simulink model "FOC_tune"  (R2022b)
settings: Solver=VariableStepAuto  StartTime=0.0  StopTime=40  RelTol=1e-3
libraries: spsMosfetLib x6, slpidlib x5, spsDCVoltageSourceLib x1, spsTriangleGeneratorLib x1, spsPermanentMagnetSynchronousMachineLib x1, spspowerguiLib x1
settings Model: Creator=ozgur  LastModifiedBy=ozgur

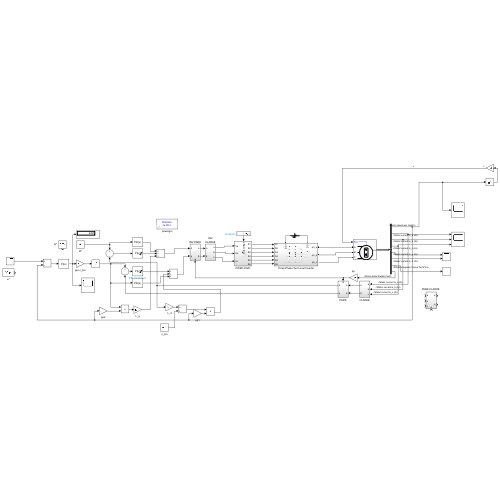
[thumbnail: Simulink's stored preview of the top-level diagram]
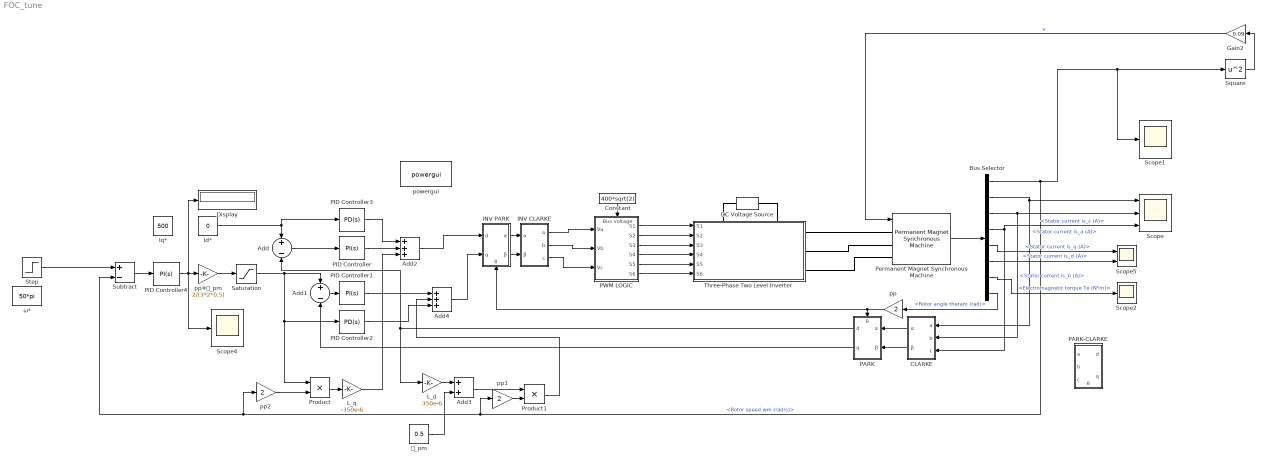
== system FOC_tune ==
  Add : Sum  Inputs=+-
  Add1 : Sum  Inputs=+-
  Add2 : Sum  Inputs=+++
  Add3 : Sum
  Add4 : Sum  Inputs=+++
  Bus Selector : BusSelector  OutputSignals=Rotor speed wm (rad/s),Stator current is_a (A),Stator current is_b (A),Stator current is_c (A),Stator current is_q (A),Stator current is_d (A),Electromagnetic torque Te (N*m),Rotor angle thetam (rad)
  CLARKE : Subsystem
  Constant : Constant  Value=400*sqrt(2)
  DC Voltage Source : spsDCVoltageSourceLib/DC Voltage Source  Amplitude=400*sqrt(2)  Measurements=None
  Display : Display
  Gain2 : Gain  Gain=0.09
  INV CLARKE : Subsystem
  INV PARK : Subsystem
      settings: PortSchema="{\"entries\":[{\"content\":{\"sides\":[{\"content\":{\"connectorIds\":[\"In1\",\"In2\"]},\"type\":\"ConnectorPlacement.EquallySpacedRectSide\",\"uuid\":\"59903cba-fdd3-44d5-a192-a04f64287d2b\"},{\"content\":{\"connectorIds\":[\"Out1\",\"Out2\"],\"side\":\"RIGHT\"},\"type\":\"ConnectorPlacement.EquallySpacedRectSide\",\"uuid\":\"681eb959-6b17-4a1b-ad29-ed5ddea04885\"},{\"content\":{\"connectorIds\":[],\"side\":\"TOP\"},\"type\":\"ConnectorPlacement.EquallySpacedRectSide\",\"uuid\":\"06ff0d1b-ee3f-4b4d-8458-3ce27937f61b\"},{\"content\":{\"connectorIds\":[\"In3\"],\"side\":\"BOTTOM\"},\"type\":\"ConnectorPlacement.EquallySpacedRectSide\",\"uuid\":\"72d471a0-f669-4f45-bd77-3491789d9278\"}]},\"type\":\"ConnectorPlacement.EquallySpacedConnector\",\"uuid\":\"36f25fd4-dcd9-497f-b503-ff3ea179f7f9\"}],\"packageUris\":[\"http://schema.mathworks.com/mf0/Connector/R2020b\"],\"version\":\"1.0\"}"
  Id* : Constant  Value=0
  Iq* : Constant  Value=500
  L_d : Gain  Gain=350e-6
  L_q : Gain  Gain=-350e-6
  PARK : Subsystem
      settings: PortSchema="{\"entries\":[{\"content\":{\"sides\":[{\"content\":{\"connectorIds\":[\"In1\",\"In2\"]},\"type\":\"ConnectorPlacement.EquallySpacedRectSide\",\"uuid\":\"59903cba-fdd3-44d5-a192-a04f64287d2b\"},{\"content\":{\"connectorIds\":[\"Out1\",\"Out2\"],\"side\":\"RIGHT\"},\"type\":\"ConnectorPlacement.EquallySpacedRectSide\",\"uuid\":\"681eb959-6b17-4a1b-ad29-ed5ddea04885\"},{\"content\":{\"connectorIds\":[],\"side\":\"TOP\"},\"type\":\"ConnectorPlacement.EquallySpacedRectSide\",\"uuid\":\"06ff0d1b-ee3f-4b4d-8458-3ce27937f61b\"},{\"content\":{\"connectorIds\":[\"In3\"],\"side\":\"BOTTOM\"},\"type\":\"ConnectorPlacement.EquallySpacedRectSide\",\"uuid\":\"f222b3cd-2ed5-40df-a353-68c0040cbc2b\"}]},\"type\":\"ConnectorPlacement.EquallySpacedConnector\",\"uuid\":\"36f25fd4-dcd9-497f-b503-ff3ea179f7f9\"}],\"packageUris\":[\"http://schema.mathworks.com/mf0/Connector/R2020b\"],\"version\":\"1.0\"}"
  "PARK-CLARKE " : Subsystem
      settings: PortSchema="{\"entries\":[{\"content\":{\"sides\":[{\"content\":{\"connectorIds\":[\"In1\",\"In2\",\"In3\"]},\"type\":\"ConnectorPlacement.EquallySpacedRectSide\",\"uuid\":\"919e8c4c-7bf6-4556-96cc-e7d0cf6a5642\"},{\"content\":{\"connectorIds\":[\"Out1\",\"Out2\"],\"side\":\"RIGHT\"},\"type\":\"ConnectorPlacement.EquallySpacedRectSide\",\"uuid\":\"e13b297b-3f4b-4600-882f-43fb25cf0d8f\"},{\"content\":{\"connectorIds\":[],\"side\":\"TOP\"},\"type\":\"ConnectorPlacement.EquallySpacedRectSide\",\"uuid\":\"2e88e734-d7e0-49ab-829a-d0bb9349cfd8\"},{\"content\":{\"connectorIds\":[\"In4\"],\"side\":\"BOTTOM\"},\"type\":\"ConnectorPlacement.EquallySpacedRectSide\",\"uuid\":\"abca995e-4a31-4078-bb38-c1490f0679d8\"}]},\"type\":\"ConnectorPlacement.EquallySpacedConnector\",\"uuid\":\"7a89cad2-f190-4924-930b-5dfa2afe5fc8\"}],\"packageUris\":[\"http://schema.mathworks.com/mf0/Connector/R2020b\"],\"version\":\"1.0\"}"
  PID Controller : slpidlib/PID Controller  Controller=PI  Form=Parallel  TimeDomain=Continuous-time  UseExternalTs=off  SampleTime=-1  IntegratorMethod=Forward Euler  FilterMethod=Forward Euler  ControllerParametersSource=internal  P=200*pi*2*350*10e-6  I=0.016*200*2*pi  UseKiTs=off  D=350e-3  N=100  UseFilter=on  TunerSelectOption=Transfer Function Based (PID Tuner App)  InitialConditionSource=internal  InitialConditionForIntegrator=0  InitialConditionForFilter=0  DifferentiatorICPrevScaledInput=0  ExternalReset=none  TrackingMode=off  Kt=1  LimitOutput=on  SatLimitsSource=internal  UpperSaturationLimit=400*sqrt(2)  LowerSaturationLimit=-400*sqrt(2)  LinearizeAsGain=on  AntiWindupMode=none  Kb=1  LimitIntegrator=off  UpperIntegratorSaturationLimit=inf  LowerIntegratorSaturationLimit=-inf  POutMin=[]  POutMax=[]  IOutMin=[]  IOutMax=[]  DOutMin=[]  DOutMax=[]  NOutMin=[]  NOutMax=[]  SumOutMin=[]  SumOutMax=[]  SaturationOutMin=[]  SaturationOutMax=[]  PParamMin=[]  PParamMax=[]  IParamMin=[]  IParamMax=[]  DParamMin=[]  DParamMax=[]  NParamMin=[]  NParamMax=[]  KbParamMin=[]  KbParamMax=[]  KtParamMin=[]  KtParamMax=[]  KbOutMin=[]  KbOutMax=[]  KtOutMin=[]  KtOutMax=[]  IntegratorOutMin=[]  IntegratorOutMax=[]  FilterOutMin=[]  FilterOutMax=[]  SumI1OutMin=[]  SumI1OutMax=[]  SumI2OutMin=[]  SumI2OutMax=[]  SumI3OutMin=[]  SumI3OutMax=[]  SumI4OutMin=[]  SumI4OutMax=[]  SumDOutMin=[]  SumDOutMax=[]  DifferentiatorOutMin=[]  DifferentiatorOutMax=[]  FilterDiffOutCoefMin=[]  FilterDiffOutCoefMax=[]  ReciprocalOutMin=[]  ReciprocalOutMax=[]  SumDenOutMin=[]  SumDenOutMax=[]  SumNumOutMin=[]  SumNumOutMax=[]  DivideOutMin=[]  DivideOutMax=[]  UdiffTsProdOutMin=[]  UdiffTsProdOutMax=[]  NTsProdOutMin=[]  NTsProdOutMax=[]  UintegralTsProdOutMin=[]  UintegralTsProdOutMax=[]  UngainTsProdOutMin=[]  UngainTsProdOutMax=[]  ClampingZeroOutDataTypeStr=Inherit: Inherit via back propagation  ClampingZeroOutMin=[]  ClampingZeroOutMax=[]  FilterDenConstantOutDataTypeStr=Inherit: Inherit via back propagation  FilterDenConstantOutMin=[]  FilterDenConstantOutMax=[]  PCopyOutDataTypeStr=Inherit: Inherit via back propagation  PCopyOutMin=[]  PCopyOutMax=[]  NCopyOutDataTypeStr=Inherit: Inherit via back propagation  NCopyOutMin=[]  NCopyOutMax=[]  IntegratorContinuousStateAttributes=''  IntegratorStateMustResolveToSignalObject=off  IntegratorRTWStateStorageClass=Auto  FilterContinuousStateAttributes=''  FilterStateMustResolveToSignalObject=off  FilterRTWStateStorageClass=Auto  ParallelPVariant=InternalParameters  IdealPVariant=Disabled  IVariant=InternalParameters  DVariant=Disabled  IntegratorVariant=Continuous  SatVariant=Enabled  AWVariant=Passthrough  PCopyVariant=Disabled  TRVariant=Disabled  FdbkBlocksVariant=Forward  IdealPFdbkVariant=Disabled  SatFdbkVariant=Disabled  DerivativeFilterVariant=Disabled  NVariant=Disabled  NCopyVariant=Disabled_SignalSpec  FilterICVariant=Disabled  IntegratorICVariant=InternalICs  ExternalResetVariant=Disabled  TRSumVariant=Passthrough  SumFdbkVariant=Disabled  SumVariant=Sum_PI  TsampFilterVariant=InternalTs  TsampNgainVariant=Passthrough  TsampIntegralVariant=Passthrough  ExternalSaturationOutDataTypeStr=Inherit: Same as second input
  PID Controller1 : slpidlib/PID Controller  Controller=PI  Form=Parallel  TimeDomain=Continuous-time  UseExternalTs=off  SampleTime=-1  IntegratorMethod=Forward Euler  FilterMethod=Forward Euler  ControllerParametersSource=internal  P=200*pi*2*350*10e-6  I=0.016*2*pi*200  UseKiTs=off  D=0  N=100  UseFilter=on  TunerSelectOption=Transfer Function Based (PID Tuner App)  InitialConditionSource=internal  InitialConditionForIntegrator=0  InitialConditionForFilter=0  DifferentiatorICPrevScaledInput=0  ExternalReset=none  TrackingMode=off  Kt=1  LimitOutput=on  SatLimitsSource=internal  UpperSaturationLimit=400*sqrt(2)  LowerSaturationLimit=-400*sqrt(2)  LinearizeAsGain=on  AntiWindupMode=none  Kb=1  LimitIntegrator=off  UpperIntegratorSaturationLimit=inf  LowerIntegratorSaturationLimit=-inf  POutMin=[]  POutMax=[]  IOutMin=[]  IOutMax=[]  DOutMin=[]  DOutMax=[]  NOutMin=[]  NOutMax=[]  SumOutMin=[]  SumOutMax=[]  SaturationOutMin=[]  SaturationOutMax=[]  PParamMin=[]  PParamMax=[]  IParamMin=[]  IParamMax=[]  DParamMin=[]  DParamMax=[]  NParamMin=[]  NParamMax=[]  KbParamMin=[]  KbParamMax=[]  KtParamMin=[]  KtParamMax=[]  KbOutMin=[]  KbOutMax=[]  KtOutMin=[]  KtOutMax=[]  IntegratorOutMin=[]  IntegratorOutMax=[]  FilterOutMin=[]  FilterOutMax=[]  SumI1OutMin=[]  SumI1OutMax=[]  SumI2OutMin=[]  SumI2OutMax=[]  SumI3OutMin=[]  SumI3OutMax=[]  SumI4OutMin=[]  SumI4OutMax=[]  SumDOutMin=[]  SumDOutMax=[]  DifferentiatorOutMin=[]  DifferentiatorOutMax=[]  FilterDiffOutCoefMin=[]  FilterDiffOutCoefMax=[]  ReciprocalOutMin=[]  ReciprocalOutMax=[]  SumDenOutMin=[]  SumDenOutMax=[]  SumNumOutMin=[]  SumNumOutMax=[]  DivideOutMin=[]  DivideOutMax=[]  UdiffTsProdOutMin=[]  UdiffTsProdOutMax=[]  NTsProdOutMin=[]  NTsProdOutMax=[]  UintegralTsProdOutMin=[]  UintegralTsProdOutMax=[]  UngainTsProdOutMin=[]  UngainTsProdOutMax=[]  ClampingZeroOutDataTypeStr=Inherit: Inherit via back propagation  ClampingZeroOutMin=[]  ClampingZeroOutMax=[]  FilterDenConstantOutDataTypeStr=Inherit: Inherit via back propagation  FilterDenConstantOutMin=[]  FilterDenConstantOutMax=[]  PCopyOutDataTypeStr=Inherit: Inherit via back propagation  PCopyOutMin=[]  PCopyOutMax=[]  NCopyOutDataTypeStr=Inherit: Inherit via back propagation  NCopyOutMin=[]  NCopyOutMax=[]  IntegratorContinuousStateAttributes=''  IntegratorStateMustResolveToSignalObject=off  IntegratorRTWStateStorageClass=Auto  FilterContinuousStateAttributes=''  FilterStateMustResolveToSignalObject=off  FilterRTWStateStorageClass=Auto  ParallelPVariant=InternalParameters  IdealPVariant=Disabled  IVariant=InternalParameters  DVariant=Disabled  IntegratorVariant=Continuous  SatVariant=Enabled  AWVariant=Passthrough  PCopyVariant=Disabled  TRVariant=Disabled  FdbkBlocksVariant=Forward  IdealPFdbkVariant=Disabled  SatFdbkVariant=Disabled  DerivativeFilterVariant=Disabled  NVariant=Disabled  NCopyVariant=Disabled_SignalSpec  FilterICVariant=Disabled  IntegratorICVariant=InternalICs  ExternalResetVariant=Disabled  TRSumVariant=Passthrough  SumFdbkVariant=Disabled  SumVariant=Sum_PI  TsampFilterVariant=InternalTs  TsampNgainVariant=Passthrough  TsampIntegralVariant=Passthrough  ExternalSaturationOutDataTypeStr=Inherit: Same as second input
  PID Controller2 : slpidlib/PID Controller  Controller=PD  Form=Parallel  TimeDomain=Continuous-time  UseExternalTs=off  SampleTime=-1  IntegratorMethod=Forward Euler  FilterMethod=Forward Euler  ControllerParametersSource=internal  P=0.016  I=1  UseKiTs=off  D=350e-6  N=100  UseFilter=on  TunerSelectOption=Transfer Function Based (PID Tuner App)  InitialConditionSource=internal  InitialConditionForIntegrator=0  InitialConditionForFilter=0  DifferentiatorICPrevScaledInput=0  ExternalReset=none  TrackingMode=off  Kt=1  LimitOutput=off  SatLimitsSource=internal  UpperSaturationLimit=inf  LowerSaturationLimit=-inf  LinearizeAsGain=on  AntiWindupMode=none  Kb=1  LimitIntegrator=off  UpperIntegratorSaturationLimit=inf  LowerIntegratorSaturationLimit=-inf  POutMin=[]  POutMax=[]  IOutMin=[]  IOutMax=[]  DOutMin=[]  DOutMax=[]  NOutMin=[]  NOutMax=[]  SumOutMin=[]  SumOutMax=[]  SaturationOutMin=[]  SaturationOutMax=[]  PParamMin=[]  PParamMax=[]  IParamMin=[]  IParamMax=[]  DParamMin=[]  DParamMax=[]  NParamMin=[]  NParamMax=[]  KbParamMin=[]  KbParamMax=[]  KtParamMin=[]  KtParamMax=[]  KbOutMin=[]  KbOutMax=[]  KtOutMin=[]  KtOutMax=[]  IntegratorOutMin=[]  IntegratorOutMax=[]  FilterOutMin=[]  FilterOutMax=[]  SumI1OutMin=[]  SumI1OutMax=[]  SumI2OutMin=[]  SumI2OutMax=[]  SumI3OutMin=[]  SumI3OutMax=[]  SumI4OutMin=[]  SumI4OutMax=[]  SumDOutMin=[]  SumDOutMax=[]  DifferentiatorOutMin=[]  DifferentiatorOutMax=[]  FilterDiffOutCoefMin=[]  FilterDiffOutCoefMax=[]  ReciprocalOutMin=[]  ReciprocalOutMax=[]  SumDenOutMin=[]  SumDenOutMax=[]  SumNumOutMin=[]  SumNumOutMax=[]  DivideOutMin=[]  DivideOutMax=[]  UdiffTsProdOutMin=[]  UdiffTsProdOutMax=[]  NTsProdOutMin=[]  NTsProdOutMax=[]  UintegralTsProdOutMin=[]  UintegralTsProdOutMax=[]  UngainTsProdOutMin=[]  UngainTsProdOutMax=[]  ClampingZeroOutDataTypeStr=Inherit: Inherit via back propagation  ClampingZeroOutMin=[]  ClampingZeroOutMax=[]  FilterDenConstantOutDataTypeStr=Inherit: Inherit via back propagation  FilterDenConstantOutMin=[]  FilterDenConstantOutMax=[]  PCopyOutDataTypeStr=Inherit: Inherit via back propagation  PCopyOutMin=[]  PCopyOutMax=[]  NCopyOutDataTypeStr=Inherit: Inherit via back propagation  NCopyOutMin=[]  NCopyOutMax=[]  IntegratorContinuousStateAttributes=''  IntegratorStateMustResolveToSignalObject=off  IntegratorRTWStateStorageClass=Auto  FilterContinuousStateAttributes=''  FilterStateMustResolveToSignalObject=off  FilterRTWStateStorageClass=Auto  ParallelPVariant=InternalParameters  IdealPVariant=Disabled  IVariant=Disabled  DVariant=InternalParameters  IntegratorVariant=Disabled  SatVariant=Disabled  AWVariant=Disabled  PCopyVariant=Disabled  TRVariant=Disabled  FdbkBlocksVariant=Forward  IdealPFdbkVariant=Disabled  SatFdbkVariant=Disabled  DerivativeFilterVariant=ContFilter  NVariant=InternalParameters  NCopyVariant=Disabled  FilterICVariant=InternalICsFilter  IntegratorICVariant=Disabled  ExternalResetVariant=Disabled  TRSumVariant=Passthrough  SumFdbkVariant=Disabled  SumVariant=Sum_PD  TsampFilterVariant=InternalTs  TsampNgainVariant=Passthrough  TsampIntegralVariant=Disabled_SignalSpec  ExternalSaturationOutDataTypeStr=Inherit: Same as second input
  PID Controller3 : slpidlib/PID Controller  Controller=PD  Form=Parallel  TimeDomain=Continuous-time  UseExternalTs=off  SampleTime=-1  IntegratorMethod=Forward Euler  FilterMethod=Forward Euler  ControllerParametersSource=internal  P=0.016  I=1  UseKiTs=off  D=350e-6  N=100  UseFilter=on  TunerSelectOption=Transfer Function Based (PID Tuner App)  InitialConditionSource=internal  InitialConditionForIntegrator=0  InitialConditionForFilter=0  DifferentiatorICPrevScaledInput=0  ExternalReset=none  TrackingMode=off  Kt=1  LimitOutput=off  SatLimitsSource=internal  UpperSaturationLimit=inf  LowerSaturationLimit=-inf  LinearizeAsGain=on  AntiWindupMode=none  Kb=1  LimitIntegrator=off  UpperIntegratorSaturationLimit=inf  LowerIntegratorSaturationLimit=-inf  POutMin=[]  POutMax=[]  IOutMin=[]  IOutMax=[]  DOutMin=[]  DOutMax=[]  NOutMin=[]  NOutMax=[]  SumOutMin=[]  SumOutMax=[]  SaturationOutMin=[]  SaturationOutMax=[]  PParamMin=[]  PParamMax=[]  IParamMin=[]  IParamMax=[]  DParamMin=[]  DParamMax=[]  NParamMin=[]  NParamMax=[]  KbParamMin=[]  KbParamMax=[]  KtParamMin=[]  KtParamMax=[]  KbOutMin=[]  KbOutMax=[]  KtOutMin=[]  KtOutMax=[]  IntegratorOutMin=[]  IntegratorOutMax=[]  FilterOutMin=[]  FilterOutMax=[]  SumI1OutMin=[]  SumI1OutMax=[]  SumI2OutMin=[]  SumI2OutMax=[]  SumI3OutMin=[]  SumI3OutMax=[]  SumI4OutMin=[]  SumI4OutMax=[]  SumDOutMin=[]  SumDOutMax=[]  DifferentiatorOutMin=[]  DifferentiatorOutMax=[]  FilterDiffOutCoefMin=[]  FilterDiffOutCoefMax=[]  ReciprocalOutMin=[]  ReciprocalOutMax=[]  SumDenOutMin=[]  SumDenOutMax=[]  SumNumOutMin=[]  SumNumOutMax=[]  DivideOutMin=[]  DivideOutMax=[]  UdiffTsProdOutMin=[]  UdiffTsProdOutMax=[]  NTsProdOutMin=[]  NTsProdOutMax=[]  UintegralTsProdOutMin=[]  UintegralTsProdOutMax=[]  UngainTsProdOutMin=[]  UngainTsProdOutMax=[]  ClampingZeroOutDataTypeStr=Inherit: Inherit via back propagation  ClampingZeroOutMin=[]  ClampingZeroOutMax=[]  FilterDenConstantOutDataTypeStr=Inherit: Inherit via back propagation  FilterDenConstantOutMin=[]  FilterDenConstantOutMax=[]  PCopyOutDataTypeStr=Inherit: Inherit via back propagation  PCopyOutMin=[]  PCopyOutMax=[]  NCopyOutDataTypeStr=Inherit: Inherit via back propagation  NCopyOutMin=[]  NCopyOutMax=[]  IntegratorContinuousStateAttributes=''  IntegratorStateMustResolveToSignalObject=off  IntegratorRTWStateStorageClass=Auto  FilterContinuousStateAttributes=''  FilterStateMustResolveToSignalObject=off  FilterRTWStateStorageClass=Auto  ParallelPVariant=InternalParameters  IdealPVariant=Disabled  IVariant=Disabled  DVariant=InternalParameters  IntegratorVariant=Disabled  SatVariant=Disabled  AWVariant=Disabled  PCopyVariant=Disabled  TRVariant=Disabled  FdbkBlocksVariant=Forward  IdealPFdbkVariant=Disabled  SatFdbkVariant=Disabled  DerivativeFilterVariant=ContFilter  NVariant=InternalParameters  NCopyVariant=Disabled  FilterICVariant=InternalICsFilter  IntegratorICVariant=Disabled  ExternalResetVariant=Disabled  TRSumVariant=Passthrough  SumFdbkVariant=Disabled  SumVariant=Sum_PD  TsampFilterVariant=InternalTs  TsampNgainVariant=Passthrough  TsampIntegralVariant=Disabled_SignalSpec  ExternalSaturationOutDataTypeStr=Inherit: Same as second input
  PID Controller4 : slpidlib/PID Controller  Controller=PI  Form=Parallel  TimeDomain=Continuous-time  UseExternalTs=off  SampleTime=-1  IntegratorMethod=Forward Euler  FilterMethod=Forward Euler  ControllerParametersSource=internal  P=241*2*pi*200/10/(3/2*2*0.5)/100  I=241*(2*pi*200/10)^2/(3/2*2*0.5*5)/10000  UseKiTs=off  D=0  N=100  UseFilter=on  TunerSelectOption=Transfer Function Based (PID Tuner App)  InitialConditionSource=internal  InitialConditionForIntegrator=0  InitialConditionForFilter=0  DifferentiatorICPrevScaledInput=0  ExternalReset=none  TrackingMode=off  Kt=1  LimitOutput=off  SatLimitsSource=internal  UpperSaturationLimit=inf  LowerSaturationLimit=-inf  LinearizeAsGain=on  AntiWindupMode=none  Kb=1  LimitIntegrator=off  UpperIntegratorSaturationLimit=inf  LowerIntegratorSaturationLimit=-inf  POutMin=[]  POutMax=[]  IOutMin=[]  IOutMax=[]  DOutMin=[]  DOutMax=[]  NOutMin=[]  NOutMax=[]  SumOutMin=[]  SumOutMax=[]  SaturationOutMin=[]  SaturationOutMax=[]  PParamMin=[]  PParamMax=[]  IParamMin=[]  IParamMax=[]  DParamMin=[]  DParamMax=[]  NParamMin=[]  NParamMax=[]  KbParamMin=[]  KbParamMax=[]  KtParamMin=[]  KtParamMax=[]  KbOutMin=[]  KbOutMax=[]  KtOutMin=[]  KtOutMax=[]  IntegratorOutMin=[]  IntegratorOutMax=[]  FilterOutMin=[]  FilterOutMax=[]  SumI1OutMin=[]  SumI1OutMax=[]  SumI2OutMin=[]  SumI2OutMax=[]  SumI3OutMin=[]  SumI3OutMax=[]  SumI4OutMin=[]  SumI4OutMax=[]  SumDOutMin=[]  SumDOutMax=[]  DifferentiatorOutMin=[]  DifferentiatorOutMax=[]  FilterDiffOutCoefMin=[]  FilterDiffOutCoefMax=[]  ReciprocalOutMin=[]  ReciprocalOutMax=[]  SumDenOutMin=[]  SumDenOutMax=[]  SumNumOutMin=[]  SumNumOutMax=[]  DivideOutMin=[]  DivideOutMax=[]  UdiffTsProdOutMin=[]  UdiffTsProdOutMax=[]  NTsProdOutMin=[]  NTsProdOutMax=[]  UintegralTsProdOutMin=[]  UintegralTsProdOutMax=[]  UngainTsProdOutMin=[]  UngainTsProdOutMax=[]  ClampingZeroOutDataTypeStr=Inherit: Inherit via back propagation  ClampingZeroOutMin=[]  ClampingZeroOutMax=[]  FilterDenConstantOutDataTypeStr=Inherit: Inherit via back propagation  FilterDenConstantOutMin=[]  FilterDenConstantOutMax=[]  PCopyOutDataTypeStr=Inherit: Inherit via back propagation  PCopyOutMin=[]  PCopyOutMax=[]  NCopyOutDataTypeStr=Inherit: Inherit via back propagation  NCopyOutMin=[]  NCopyOutMax=[]  IntegratorContinuousStateAttributes=''  IntegratorStateMustResolveToSignalObject=off  IntegratorRTWStateStorageClass=Auto  FilterContinuousStateAttributes=''  FilterStateMustResolveToSignalObject=off  FilterRTWStateStorageClass=Auto  ParallelPVariant=InternalParameters  IdealPVariant=Disabled  IVariant=InternalParameters  DVariant=Disabled  IntegratorVariant=Continuous  SatVariant=Disabled  AWVariant=Passthrough  PCopyVariant=Disabled  TRVariant=Disabled  FdbkBlocksVariant=Forward  IdealPFdbkVariant=Disabled  SatFdbkVariant=Disabled  DerivativeFilterVariant=Disabled  NVariant=Disabled  NCopyVariant=Disabled_SignalSpec  FilterICVariant=Disabled  IntegratorICVariant=InternalICs  ExternalResetVariant=Disabled  TRSumVariant=Passthrough  SumFdbkVariant=Disabled  SumVariant=Sum_PI  TsampFilterVariant=InternalTs  TsampNgainVariant=Passthrough  TsampIntegralVariant=Passthrough  ExternalSaturationOutDataTypeStr=Inherit: Same as second input
  PWM LOGIC : Subsystem
      settings: PortSchema="{\"entries\":[{\"content\":{\"sides\":[{\"content\":{\"connectorIds\":[\"In1\",\"In2\",\"In3\"]},\"type\":\"ConnectorPlacement.EquallySpacedRectSide\",\"uuid\":\"1ce4e2f6-7038-429d-a80c-8e15bf83e4cb\"},{\"content\":{\"connectorIds\":[\"Out1\",\"Out2\",\"Out3\",\"Out4\",\"Out5\",\"Out6\"],\"side\":\"RIGHT\"},\"type\":\"ConnectorPlacement.EquallySpacedRectSide\",\"uuid\":\"9e66ec41-835d-4e36-a70d-c94b943e8eb4\"},{\"content\":{\"connectorIds\":[\"In4\"],\"side\":\"TOP\"},\"type\":\"ConnectorPlacement.EquallySpacedRectSide\",\"uuid\":\"ff913cb9-b27a-4317-8890-2abc2a2b35df\"}]},\"type\":\"ConnectorPlacement.EquallySpacedConnector\",\"uuid\":\"023ac905-18b6-49df-b833-53e972ba8e5b\"}],\"packageUris\":[\"http://schema.mathworks.com/mf0/Connector/R2020b\"],\"version\":\"1.0\"}"
  Permanent Magnet Synchronous Machine : spsPermanentMagnetSynchronousMachineLib/Permanent Magnet Synchronous Machine  NbPhases=3  FluxDistribution=Sinusoidal  RotorType=Round  MechanicalLoad=Torque Tm  PresetModel=No  ShowDetailedParameters=on  MeasurementBus=off  Resistance=0.016  Inductance=8.5e-3  dqInductances=[8.5e-3,8.5e-3]  La=350e-6  MachineConstant=Flux linkage established by magnets (V.s)  Flux=0.5  VoltageCst=181.3799  TorqueCst=1.5  Flat=120  Mechanical=[241 0 2 0]  PolePairs=4  InitialConditions=[45*pi,0, 0, 0]  InitialConditions5ph=[0 0 0 0 0 0]  RefAngle=Aligned with phase A axis (original Park)  IterativeDiscreteModel=Trapezoidal non iterative  TsBlock=-1  TsPowergui=0
  Product : Product
  Product1 : Product
  Saturation : Saturate  UpperLimit=3400  LowerLimit=-3400
  Scope : Scope  NumInputPorts=3
  Scope1 : Scope
  Scope2 : Scope
  Scope4 : Scope
  Scope5 : Scope  NumInputPorts=2
  Square : Math  Operator=square
  Step : Step  Time=10  Before=45*pi  After=50*pi  SampleTime=0
  Subtract : Sum  Inputs=+-
  Three-Phase Two Level Inverter : Subsystem
      settings: PortSchema="{\"entries\":[{\"content\":{\"sides\":[{\"content\":{\"connectorIds\":[\"In1\",\"In2\",\"In3\",\"In4\",\"In5\",\"In6\"]},\"type\":\"ConnectorPlacement.EquallySpacedRectSide\",\"uuid\":\"f37396d3-5f1b-4e56-a823-dcd858233f1a\"},{\"content\":{\"connectorIds\":[\"RConn1\",\"RConn2\",\"RConn3\"],\"side\":\"RIGHT\"},\"type\":\"ConnectorPlacement.EquallySpacedRectSide\",\"uuid\":\"1e664dad-64e8-4dd7-b45b-69867f9f15f6\"},{\"content\":{\"connectorIds\":[\"LConn1\",\"LConn2\"],\"side\":\"TOP\"},\"type\":\"ConnectorPlacement.EquallySpacedRectSide\",\"uuid\":\"e8259c77-b4f1-49c6-8925-8fb334cba9ae\"}]},\"type\":\"ConnectorPlacement.EquallySpacedConnector\",\"uuid\":\"1b57e49d-21de-45ee-b574-b0ea2af2b502\"}],\"packageUris\":[\"http://schema.mathworks.com/mf0/Connector/R2020b\"],\"version\":\"1.0\"}"
  powergui : spspowerguiLib/powergui  Priority=1  SimulationMode=Discrete  SampleTime=10e-6  frequency=60  Iterations=50  frequencyindice=0  Pbase=100e6  ErrMax=1e-4  UnitsV=kV  UnitsW=MW  buscounter=0  FunctionMessages=off  echomessages=off  EnableUseOfTLC=off  CurrentSourceSwitches=off  DisableSnubberDevices=off  DisableRonSwitches=off  DisableVfSwitches=off  DisplayEquations=off  AutomaticDiscreteSolvers=off  SolverType=Tustin/Backward Euler (TBE)  Interpol=off  ExternalGateDelay=off  methode=off  Ts=100  x0status=blocks  SPID=on  SwTol=0  HookPort=off  NonlinearTolerance=1e-4  nMaxIteration=100  ContinueOnMaxIteration=off  RestoreLinks=warning  ResistiveCurrentMeasurement=off  Frange=[0:2:500]  Ylog=off  Xlog=on  ShowGrid=off  save=off  variable=ZData  structure=0  ZoomFFT=off  StartTime=0.0  cycles=1  DisplayStyle=1  fundamental=60  FreqAxis=off  MaxFrequency=1000  frequencyindicesteady=1  RmsSteady=1  display=off
  pp : Gain  Gain=2
  pp+𝜆_pm : Gain  Gain=2/(3*2*0.5)
  pp1 : Gain  Gain=2
  pp2 : Gain  Gain=2
  ω* : Constant  Value=50*pi
  𝜆_pm : Constant  Value=0.5
  wires:
  Permanent Magnet Synchronous Machine/1 -> Bus Selector/1
  Bus Selector/4 -> Scope/3, CLARKE/3(c)  "<Stator current is_c (A)>"
  Bus Selector/3 -> Scope/2, CLARKE/2(b)  "<Stator current is_b (A)>"
  Bus Selector/2 -> CLARKE/1(a), Scope/1  "<Stator current is_a (A)>"
  CLARKE/1(α) -> PARK/2(α)
  CLARKE/2(β) -> PARK/1(β)
  Bus Selector/8 -> pp/1  "<Rotor angle thetam (rad)>"
  PARK/2(d) -> L_d/1, Add/2
  Id*/1 -> PID Controller3/1, Add/1
  Add/1 -> PID Controller/1
  PARK/1(q) -> Add1/2
  PID Controller/1 -> Add2/2
  Product/1 -> L_q/1
  L_q/1 -> Add2/3
  Add2/1 -> INV PARK/1(d)
  INV PARK/1(α) -> INV CLARKE/1(α)
  INV PARK/2(β) -> INV CLARKE/2(β)
  INV CLARKE/1(a) -> PWM LOGIC/1(Va)
  INV CLARKE/2(b) -> PWM LOGIC/2(Vb)
  INV CLARKE/3(c) -> PWM LOGIC/3(Vc)
  PWM LOGIC/4(S4) -> Three-Phase Two Level Inverter/4(S4)
  PWM LOGIC/3(S3) -> Three-Phase Two Level Inverter/3(S3)
  PWM LOGIC/2(S2) -> Three-Phase Two Level Inverter/2(S2)
  PWM LOGIC/1(S1) -> Three-Phase Two Level Inverter/1(S1)
  PWM LOGIC/6(S6) -> Three-Phase Two Level Inverter/6(S6)
  PWM LOGIC/5(S5) -> Three-Phase Two Level Inverter/5(S5)
  L_d/1 -> Add3/1
  𝜆_pm/1 -> Add3/2
  Add3/1 -> Product1/1
  Add1/1 -> PID Controller1/1
  Add4/1 -> INV PARK/2(q)
  PID Controller1/1 -> Add4/1
  Product1/1 -> Add4/2
  PID Controller2/1 -> Add4/3
  PID Controller3/1 -> Add2/1
  Constant/1 -> PWM LOGIC/4(Bus voltage)
  Bus Selector/1 -> Scope1/1, Square/1, pp1/1, pp2/1, Subtract/2  "<Rotor speed wm (rad/s)>"
  Gain2/1 -> Permanent Magnet Synchronous Machine/1  "v"
  Square/1 -> Gain2/1
  Saturation/1 -> PID Controller2/1, Product/1, Add1/1
  PID Controller4/1 -> Display/1, Scope4/1, pp+𝜆_pm/1
  Subtract/1 -> PID Controller4/1
  Bus Selector/7 -> Scope2/1  "<Electromagnetic torque Te (N*m)>"
  pp/1 -> INV PARK/3(θ), PARK/3(θ)
  pp1/1 -> Product1/2
  pp2/1 -> Product/2
  Step/1 -> Subtract/1
  Bus Selector/5 -> Scope5/1  "<Stator current is_q (A)>"
  Bus Selector/6 -> Scope5/2  "<Stator current is_d (A)>"
  pp+𝜆_pm/1 -> Saturation/1
  connections:
  DC Voltage Source/RConn1 -- Three-Phase Two Level Inverter/LConn1
  DC Voltage Source/LConn1 -- Three-Phase Two Level Inverter/LConn2
  Three-Phase Two Level Inverter/RConn1 -- Permanent Magnet Synchronous Machine/LConn1
  Three-Phase Two Level Inverter/RConn2 -- Permanent Magnet Synchronous Machine/LConn2
  Three-Phase Two Level Inverter/RConn3 -- Permanent Magnet Synchronous Machine/LConn3

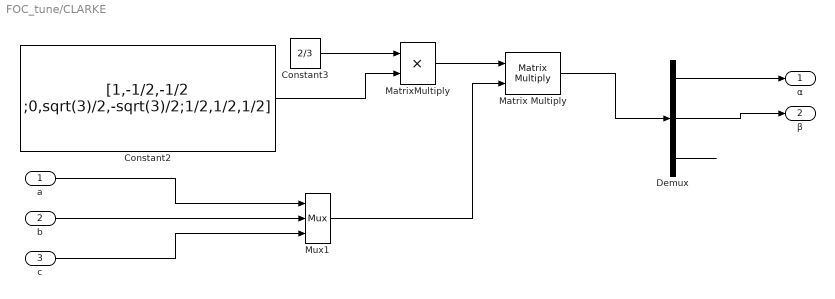
== system FOC_tune/CLARKE ==
  a : Inport
  b : Inport  Port=2
  c : Inport  Port=3
  Constant2 : Constant  Value=[1,-1/2,-1/2 ;0,sqrt(3)/2,-sqrt(3)/2;1/2,1/2,1/2]  VectorParams1D=off
  Constant3 : Constant  Value=2/3
  Demux : Demux  Outputs=3
  Matrix Multiply : Product  Multiplication=Matrix(*)
  MatrixMultiply : Product
  Mux1 : Mux  Inputs=3
  α : Outport
  β : Outport  Port=2
  wires:
  Matrix Multiply/1 -> Demux/1
  a/1 -> Mux1/1
  MatrixMultiply/1 -> Matrix Multiply/1
  Mux1/1 -> Matrix Multiply/2
  c/1 -> Mux1/3
  Demux/1 -> α/1
  Constant3/1 -> MatrixMultiply/1
  b/1 -> Mux1/2
  Constant2/1 -> MatrixMultiply/2
  Demux/2 -> β/1
  Demux/3 -> ?

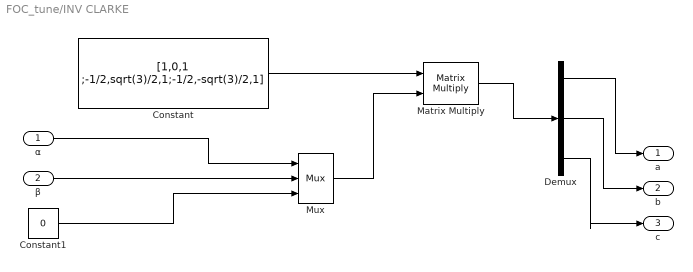
== system FOC_tune/INV CLARKE ==
  α : Inport
  β : Inport  Port=2
  Constant : Constant  Value=[1,0,1 ;-1/2,sqrt(3)/2,1;-1/2,-sqrt(3)/2,1]  VectorParams1D=off
  Constant1 : Constant  Value=0
  Demux : Demux  Outputs=3
  Matrix Multiply : Product  Multiplication=Matrix(*)
  Mux : Mux  Inputs=3
  a : Outport
  b : Outport  Port=2
  c : Outport  Port=3
  wires:
  Matrix Multiply/1 -> Demux/1
  Demux/2 -> b/1
  Demux/1 -> a/1
  α/1 -> Mux/1
  Demux/3 -> c/1
  Constant1/1 -> Mux/3
  Constant/1 -> Matrix Multiply/1
  β/1 -> Mux/2
  Mux/1 -> Matrix Multiply/2

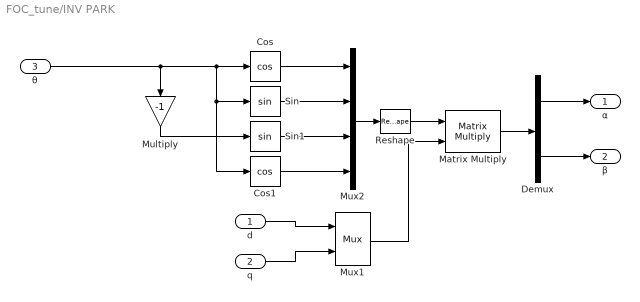
== system FOC_tune/INV PARK ==
  d : Inport
  q : Inport  Port=2
  θ : Inport  Port=3
  Cos : Trigonometry  Operator=cos
  Cos1 : Trigonometry  Operator=cos
  Demux : Demux  Outputs=2
  Matrix Multiply : Product  Multiplication=Matrix(*)
  Multiply : Gain  Gain=-1
  Mux1 : Mux  Inputs=2
  Mux2 : Mux
  Reshape : Reshape  OutputDimensionality=Customize  OutputDimensions=[2,2]
  Sin : Trigonometry
  Sin1 : Trigonometry
  α : Outport
  β : Outport  Port=2
  wires:
  Sin1/1 -> Mux2/3
  Matrix Multiply/1 -> Demux/1
  Sin/1 -> Mux2/2
  d/1 -> Mux1/1
  Reshape/1 -> Matrix Multiply/1
  θ/1 -> Cos/1, Cos1/1, Sin/1, Multiply/1
  Cos1/1 -> Mux2/4
  Demux/2 -> β/1
  q/1 -> Mux1/2
  Demux/1 -> α/1
  Mux1/1 -> Matrix Multiply/2
  Cos/1 -> Mux2/1
  Mux2/1 -> Reshape/1
  Multiply/1 -> Sin1/1

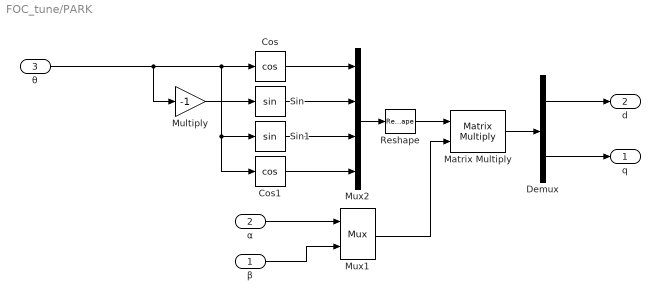
== system FOC_tune/PARK ==
  β : Inport
  α : Inport  Port=2
  θ : Inport  Port=3
  Cos : Trigonometry  Operator=cos
  Cos1 : Trigonometry  Operator=cos
  Demux : Demux  Outputs=2
  Matrix Multiply : Product  Multiplication=Matrix(*)
  Multiply : Gain  Gain=-1
  Mux1 : Mux  Inputs=2
  Mux2 : Mux
  Reshape : Reshape  OutputDimensionality=Customize  OutputDimensions=[2,2]
  Sin : Trigonometry
  Sin1 : Trigonometry
  q : Outport
  d : Outport  Port=2
  wires:
  Cos1/1 -> Mux2/4
  Sin/1 -> Mux2/2
  Multiply/1 -> Sin/1
  α/1 -> Mux1/1
  Demux/1 -> d/1
  Mux1/1 -> Matrix Multiply/2
  Mux2/1 -> Reshape/1
  β/1 -> Mux1/2
  θ/1 -> Cos/1, Sin1/1, Cos1/1, Multiply/1
  Matrix Multiply/1 -> Demux/1
  Reshape/1 -> Matrix Multiply/1
  Sin1/1 -> Mux2/3
  Cos/1 -> Mux2/1
  Demux/2 -> q/1

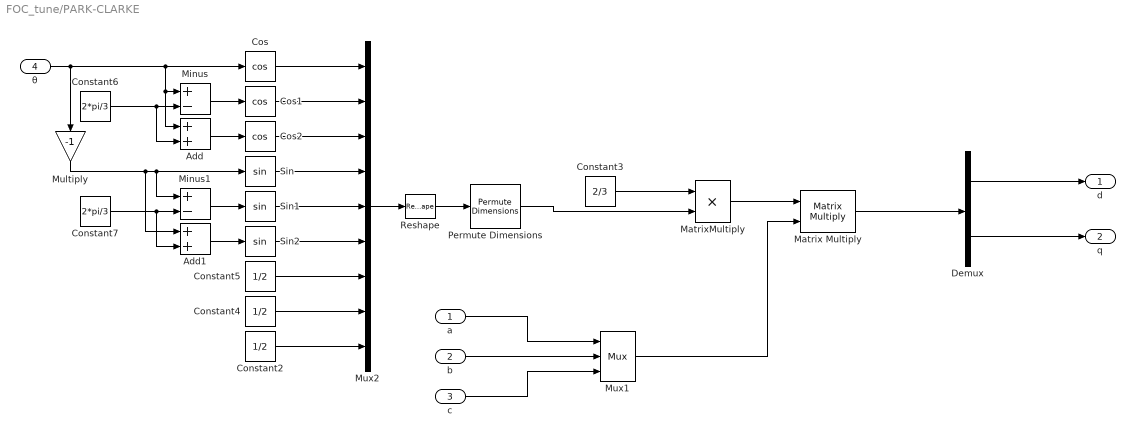
== system FOC_tune/PARK-CLARKE  ==
  a : Inport
  b : Inport  Port=2
  c : Inport  Port=3
  θ : Inport  Port=4
  Add : Sum
  Add1 : Sum
  Constant2 : Constant  Value=1/2
  Constant3 : Constant  Value=2/3
  Constant4 : Constant  Value=1/2
  Constant5 : Constant  Value=1/2
  Constant6 : Constant  Value=2*pi/3
  Constant7 : Constant  Value=2*pi/3
  Cos : Trigonometry  Operator=cos
  Cos1 : Trigonometry  Operator=cos
  Cos2 : Trigonometry  Operator=cos
  Demux : Demux  Outputs=2
  Matrix Multiply : Product  Multiplication=Matrix(*)
  MatrixMultiply : Product
  Minus : Sum  Inputs=+-
  Minus1 : Sum  Inputs=+-
  Multiply : Gain  Gain=-1
  Mux1 : Mux  Inputs=3
  Mux2 : Mux  Inputs=9
  Permute Dimensions : PermuteDimensions
  Reshape : Reshape  OutputDimensionality=Customize  OutputDimensions=[3,3]
  Sin : Trigonometry
  Sin1 : Trigonometry
  Sin2 : Trigonometry
  d : Outport
  q : Outport  Port=2
  wires:
  Constant6/1 -> Add/2, Minus/2
  θ/1 -> Cos/1, Add/1, Minus/1, Multiply/1
  Cos2/1 -> Mux2/3
  c/1 -> Mux1/3
  Constant7/1 -> Add1/2, Minus1/2
  Minus1/1 -> Sin1/1
  Sin/1 -> Mux2/4
  Cos/1 -> Mux2/1
  Permute Dimensions/1 -> MatrixMultiply/2
  b/1 -> Mux1/2
  Mux1/1 -> Matrix Multiply/2
  Constant2/1 -> Mux2/9
  Sin2/1 -> Mux2/6
  Minus/1 -> Cos1/1
  Sin1/1 -> Mux2/5
  a/1 -> Mux1/1
  Mux2/1 -> Reshape/1
  MatrixMultiply/1 -> Matrix Multiply/1
  Demux/2 -> q/1
  Add/1 -> Cos2/1
  Reshape/1 -> Permute Dimensions/1
  Constant5/1 -> Mux2/7
  Constant3/1 -> MatrixMultiply/1
  Matrix Multiply/1 -> Demux/1
  Demux/1 -> d/1
  Add1/1 -> Sin2/1
  Cos1/1 -> Mux2/2
  Constant4/1 -> Mux2/8
  Multiply/1 -> Add1/1, Minus1/1, Sin/1

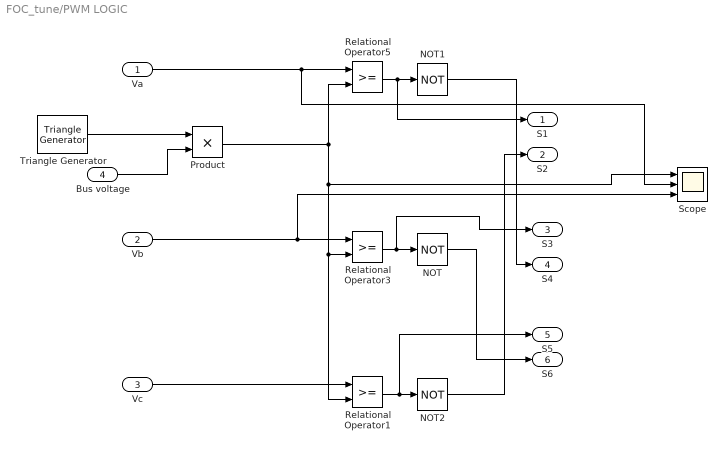
== system FOC_tune/PWM LOGIC ==
  Va : Inport
  Vb : Inport  Port=2
  Vc : Inport  Port=3
  Bus voltage : Inport  Port=4
  NOT : Logic  Operator=NOT  IconShape=distinctive  AllPortsSameDT=off  OutDataTypeStr=boolean
  NOT1 : Logic  Operator=NOT  IconShape=distinctive  AllPortsSameDT=off  OutDataTypeStr=boolean
  NOT2 : Logic  Operator=NOT  IconShape=distinctive  AllPortsSameDT=off  OutDataTypeStr=boolean
  Product : Product
  Relational Operator1 : RelationalOperator  OutDataTypeStr=boolean  RndMeth=Simplest  InputSameDT=off
  Relational Operator3 : RelationalOperator  OutDataTypeStr=boolean  RndMeth=Simplest  InputSameDT=off
  Relational Operator5 : RelationalOperator  OutDataTypeStr=boolean  RndMeth=Simplest  InputSameDT=off
  Scope : Scope  NumInputPorts=3
  Triangle Generator : spsTriangleGeneratorLib/Triangle Generator  Freq=5.1e3  Phase=0  Ts=0
  S1 : Outport
  S2 : Outport  Port=2
  S3 : Outport  Port=3
  S4 : Outport  Port=4
  S5 : Outport  Port=5
  S6 : Outport  Port=6
  wires:
  Relational Operator1/1 -> S5/1, NOT2/1
  Relational Operator5/1 -> S1/1, NOT1/1
  Vc/1 -> Relational Operator1/1
  NOT1/1 -> S4/1
  NOT2/1 -> S2/1
  NOT/1 -> S6/1
  Product/1 -> Relational Operator5/2, Relational Operator1/2, Relational Operator3/2, Scope/1
  Va/1 -> Scope/2, Relational Operator5/1
  Relational Operator3/1 -> S3/1, NOT/1
  Vb/1 -> Scope/3, Relational Operator3/1
  Triangle Generator/1 -> Product/1
  Bus voltage/1 -> Product/2

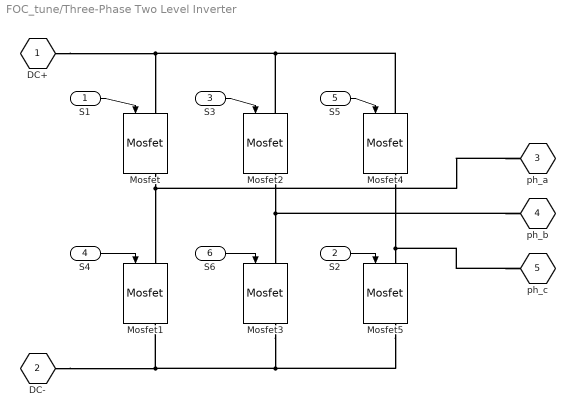
== system FOC_tune/Three-Phase Two Level Inverter ==
  S1 : Inport
  S2 : Inport  Port=2
  S3 : Inport  Port=3
  S4 : Inport  Port=4
  S5 : Inport  Port=5
  S6 : Inport  Port=6
  Mosfet{,1..5} (6 alike) : spsMosfetLib/Mosfet  Ron=0.00001  Lon=0  Rd=0.00001  Vfd=0  IC=0  Rs=1e5  Cs=inf  Measurements=on
  DC+ : PMIOPort  Side=Left
  DC- : PMIOPort  Port=2  Side=Left
  ph_a : PMIOPort  Port=3  Side=Right
  ph_b : PMIOPort  Port=4  Side=Right
  ph_c : PMIOPort  Port=5  Side=Right
  wires:
  S3/1 -> Mosfet2/1
  S5/1 -> Mosfet4/1
  S6/1 -> Mosfet3/1
  S4/1 -> Mosfet1/1
  S1/1 -> Mosfet/1
  S2/1 -> Mosfet5/1
  connections:
  Mosfet/RConn1 -- ph_a/RConn1 -- Mosfet1/LConn1
  Mosfet5/LConn1 -- Mosfet4/RConn1 -- ph_c/RConn1
  Mosfet2/LConn1 -- Mosfet4/LConn1 -- DC+/RConn1 -- Mosfet/LConn1
  Mosfet3/RConn1 -- Mosfet5/RConn1 -- DC-/RConn1 -- Mosfet1/RConn1
  Mosfet2/RConn1 -- ph_b/RConn1 -- Mosfet3/LConn1
